simulink model "OneFour3_block"  (R2022b)
settings: Solver=VariableStepAuto  StartTime=0.0  StopTime=10.0  RelTol=1e-3
settings Model: Creator=yeyi5  LastModifiedBy=yeyi5

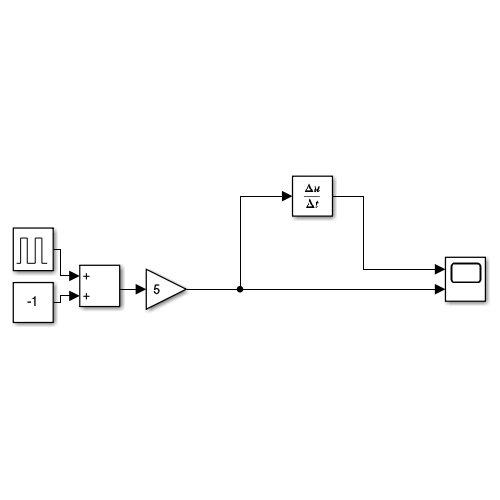
[thumbnail: Simulink's stored preview of the top-level diagram]
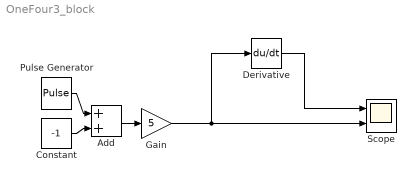
== system OneFour3_block ==
  Add : Sum
  Constant : Constant  Value=-1
  Derivative : Derivative
  Gain : Gain  Gain=5
  Pulse Generator : DiscretePulseGenerator  PulseType=Time based  Amplitude=2  Period=1/0.5  PulseWidth=50
  Scope : Scope  NumInputPorts=2
  wires:
  Derivative/1 -> Scope/1
  Pulse Generator/1 -> Add/1
  Add/1 -> Gain/1
  Constant/1 -> Add/2
  Gain/1 -> Scope/2, Derivative/1
